simulink model "mtq_allocator_unit_test"  (R2018b)
settings: Solver=VariableStepAuto  StartTime=0.0  StopTime=10.0  RelTol=1e-3
settings Model: Creator=Nick's PC  LastModifiedBy=Nick's PC

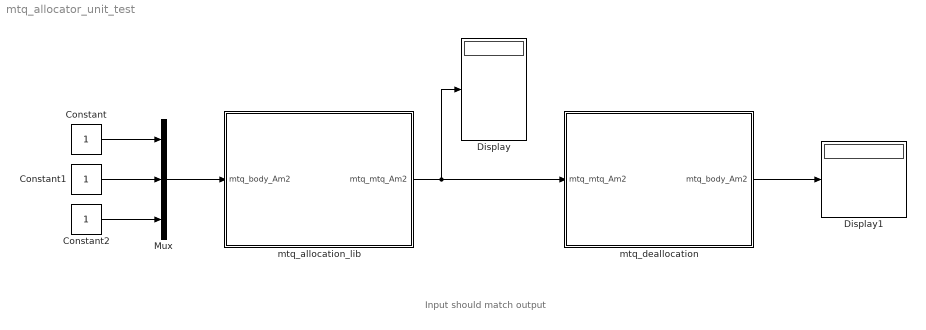
== system mtq_allocator_unit_test ==
  note: Input should match output
  Constant : Constant
  Constant1 : Constant
  Constant2 : Constant
  Display : Display
  Display1 : Display
  Mux : Mux  Inputs=3
  mtq_allocation_lib : Subsystem
  mtq_deallocation : Subsystem
  wires:
  Constant/1 -> Mux/1
  Constant1/1 -> Mux/2
  Constant2/1 -> Mux/3
  Mux/1 -> mtq_allocation_lib/1(mtq_body_Am2)
  mtq_allocation_lib/1(mtq_mtq_Am2) -> mtq_deallocation/1(mtq_mtq_Am2), Display/1
  mtq_deallocation/1(mtq_body_Am2) -> Display1/1

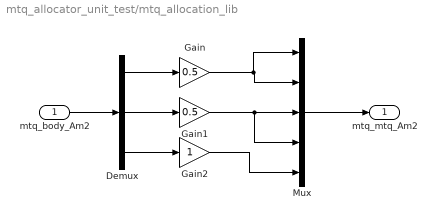
== system mtq_allocator_unit_test/mtq_allocation_lib ==
  mtq_body_Am2 : Inport
  Demux : Demux  Outputs=3
  Gain : Gain  Gain=0.5
  Gain1 : Gain  Gain=0.5
  Gain2 : Gain
  Mux : Mux  Inputs=5
  mtq_mtq_Am2 : Outport
  wires:
  mtq_body_Am2/1 -> Demux/1
  Demux/1 -> Gain/1
  Demux/2 -> Gain1/1
  Demux/3 -> Gain2/1
  Mux/1 -> mtq_mtq_Am2/1
  Gain2/1 -> Mux/5
  Gain1/1 -> Mux/3, Mux/4
  Gain/1 -> Mux/1, Mux/2

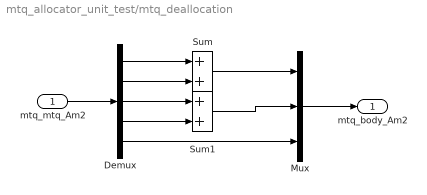
== system mtq_allocator_unit_test/mtq_deallocation ==
  mtq_mtq_Am2 : Inport
  Demux : Demux  Outputs=5
  Mux : Mux  Inputs=3
  Sum : Sum
  Sum1 : Sum
  mtq_body_Am2 : Outport
  wires:
  mtq_mtq_Am2/1 -> Demux/1
  Mux/1 -> mtq_body_Am2/1
  Demux/1 -> Sum/1
  Demux/2 -> Sum/2
  Demux/3 -> Sum1/1
  Demux/4 -> Sum1/2
  Sum/1 -> Mux/1
  Sum1/1 -> Mux/2
  Demux/5 -> Mux/3
